simulink model "ex2_model"  (R2015b)
settings: Solver=FixedStepAuto  StartTime=0.0  StopTime=5  FixedStep=0.1  RelTol=1e-3
values from neighbouring files (symbols this model uses):
  a = A(i)    [ex2_script.m]
  b = B(j)    [ex2_script.m]
settings Model: Creator=Tomáš  LastModifiedBy=Tomáš

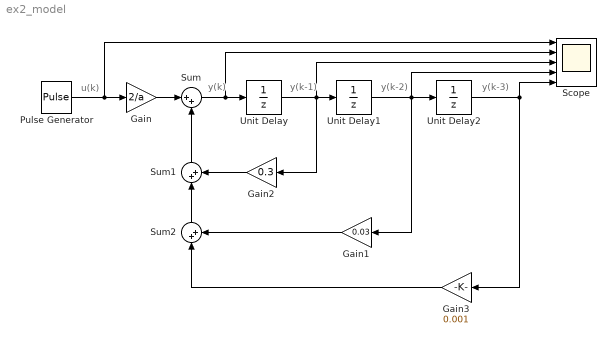
== system ex2_model ==
  note: y(k-3)
  note: y(k-2)
  note: y(k-1)
  note: y(k)
  note: u(k)
  Gain : Gain  Gain=2/a
  Gain1 : Gain  Gain=0.03
  Gain2 : Gain  Gain=0.3
  Gain3 : Gain  Gain=0.001
  Pulse Generator : DiscretePulseGenerator  PulseType=Time based  Period=1  PulseWidth=50
  Scope : Scope  NumInputPorts=5
  Sum : Sum  Inputs=|++
  Sum1 : Sum  Inputs=|++
  Sum2 : Sum  Inputs=|++
  Unit Delay : UnitDelay  InitialCondition=b  SampleTime=0.1
  Unit Delay1 : UnitDelay  InitialCondition=2*b  SampleTime=0.1
  Unit Delay2 : UnitDelay  InitialCondition=3*b  SampleTime=0.1
  wires:
  Sum/1 -> Scope/2, Unit Delay/1
  Unit Delay/1 -> Scope/3, Gain2/1, Unit Delay1/1
  Unit Delay1/1 -> Scope/4, Gain1/1, Unit Delay2/1
  Sum1/1 -> Sum/2
  Pulse Generator/1 -> Scope/1, Gain/1
  Gain/1 -> Sum/1
  Gain2/1 -> Sum1/2
  Gain1/1 -> Sum2/2
  Sum2/1 -> Sum1/1
  Gain3/1 -> Sum2/1
  Unit Delay2/1 -> Gain3/1, Scope/5
